simulink model "CompleteEngineModel_turbo"  (R2020a)
settings: Solver=ode23tb  StartTime=0  StopTime=600  MaxStep=0.4  RelTol=1e-6  AbsTol=1e-6  EnableMultiTasking=on
values from neighbouring files (symbols this model uses):
  A_eff_const = inv(A'*A)*A'*B    [Init_Project1.m]
  A_max_wg = 0.035^2/4*pi    (= 0.000962112750162)    [Init_Project1.m]    (also in Project2B.m = 0.000314159265359)
  AFs = EngineMap.airfuel.AFs    [Init_Project1.m]    (also in Project1b.m = 14)
  alpha_REF_manual = 0    [Init_Project1.m]    (also in Project2B.m)
  alphaEND = alphaINI    (= 0)    [Init_Project1.m]
  alphaINI = 0.0    (= 0)    [Init_Project1.m]
  alphaST = 30    [Init_Project1.m]
  Boost_control = 0    [Init_Project1.m]    (also in Project2B.m = 1)
  BSR_max = k(2)    [Project2A.m]
  C_d = x(3)    [Init_Project1.m]
  C_P0 = k(1)    [Project2A.m]
  C_P1 = k(2)    [Project2A.m]
  c_r1 = x(1)    [Init_Project1.m]
  c_r2 = x(2)    [Init_Project1.m]
  c_tc_fric = 1e-6    (= 1e-06)    [Init_Project1.m]    (also in Project2B.m)
  Cd_wg = 0.8    [Init_Project1.m]    (also in Project2B.m = 0.9)
  cp_air = gamma_air*cv_air    [Init_Project1.m]    (also in Project2A.m = 980)
  cp_exh = gamma_exh*cv_exh    [Init_Project1.m]    (also in Project2A.m = 1213.3)
  dP_thrREF = 10e3    (= 10000)    [Project2B.m]
  eta_c_max = k(1)    [Project2A.m]
  eta_t_max = k(1)    [Project2A.m]
  eta_vol_model = Intake_mainfold_const(1) + Intake_mainfold_const(2).*sqrt(p_im) + Intake_mainfold_const(3).*sqrt(N)    [Init_Project1.m]
  etaCmin = min(etaC/2)    [Project2A.m]
  etaTmin = min(turb.etaT)/2    [Project2A.m]
  Exhaust_flow_const = inv(A'*A)*A'*B    [Init_Project1.m]
  FMEP_const = inv(A'*A)*A'*B    [Init_Project1.m]
  Fuel_injection_const = inv(A'*A)*A'*B    [Init_Project1.m]
  gamma_air = EngineMap.airfuel.gamma_air    [Init_Project1.m]    (also in Project2A.m = 1.4)
  gamma_exh = EngineMap.airfuel.gamma_exh    [Init_Project1.m]    (also in Project2A.m = 1.3)
  Intake_mainfold_const = inv(A'*A)*A'*B    [Init_Project1.m]
  J_tc = 2.55e-5    (= 2.55e-05)    [Init_Project1.m]    (also in Project2B.m = 1e-05)
  k_0 = k(1)    [Project2A.m]
  k_1 = k(2)    [Project2A.m]
  KiDriver = 0.02    [Init_Project1.m]    (also in Project2B.m = 0.05)
  KpDriver = 0.04    [Init_Project1.m]    (also in Project2B.m = 0.8)
  KpThr = 1e-6    (= 1e-06)    [Init_Project1.m]    (also in Project2B.m)
  KpWg = 1e-6    (= 1e-06)    [Init_Project1.m]    (also in Project2B.m = 5e-06)
  m_dot_c_Corr_at = k(2)    [Project2A.m]
  m_dot_cCorr_max = k(2)    [Project2A.m]
  n_cyl = EngineMap.engine.n_cyl    [Init_Project1.m]    (also in Project2A.m)
  N_e_manual = 0    [Init_Project1.m]    (also in Project2B.m = 1)
  N_e_step = 1    [Init_Project1.m]    (also in Project2B.m)
  n_r = EngineMap.engine.n_r    [Init_Project1.m]    (also in Project2A.m; Project2B.m = 2)
  NEND = NINI    (= 2000)    [Init_Project1.m]    (also in Project2B.m = 2500)
  NeRampInit = 800    [Init_Project1.m]    (also in Project2B.m)
  NeSlope = 1    [Init_Project1.m]    (also in Project2B.m)
  NeST = 30    [Init_Project1.m]
  NINI = 2000    [Init_Project1.m]    (also in Project2B.m = 2500)
  p01 = comp.p01    [Project2A.m]
  p_amb = max(EngineMap.p_af)    [Init_Project1.m]
  pCref = comp.pCref    [Project2A.m]
  pedEND = 1.0    (= 1)    [Init_Project1.m]    (also in Project2B.m)
  pedINI = 0.2    [Init_Project1.m]    (also in Project2B.m = 0)
  pedPos_manual = 0    [Init_Project1.m]    (also in Project2B.m = 1)
  pedST = 30    [Init_Project1.m]    (also in Project2B.m)
  PiC_at = k(3)    [Project2A.m]
  Psi_max = k(1)    [Project2A.m]
  Q11 = k(4)    [Project2A.m]
  Q12 = k(5)    [Project2A.m]
  Q22 = k(6)    [Project2A.m]
  q_LHV = EngineMap.airfuel.q_LHV    [Init_Project1.m]
  R_air = EngineMap.airfuel.R_air    [Init_Project1.m]
  r_c = EngineMap.engine.r_c    [Init_Project1.m]    (also in Project1b.m = pCylHigh.r_c)
  R_exh = EngineMap.airfuel.R_exh    [Init_Project1.m]
  rComp = dComp/2    (= 0.028)    [Project2A.m]
  rho_air = p_amb/(R_air*T_amb)    [Init_Project1.m]
  rTurb = dTurb/2    (= 0.0261)    [Project2A.m]
  T01 = comp.T01    [Project2A.m]
  T_amb = mean(EngineMap.T_af)    [Init_Project1.m]
  T_bef_thr = EngineMap.T_bef_thr    [Init_Project1.m]
  T_es = EngineMap.T_es    [Init_Project1.m]
  T_ic = mean(T_bef_thr)    [Init_Project1.m]    (also in Project2B.m = T_im)
  T_im = EngineMap.T_im    [Init_Project1.m]    (also in Project1b.m = pCylHigh.T_im)
  tau_d = 0.069    [Init_Project1.m]
  tau_mix = 0.085    [Init_Project1.m]
  tau_th = 0.04    [Init_Project1.m]
  tau_wg = 0.1    [Init_Project1.m]    (also in Project2B.m)
  TCref = comp.TCref    [Project2A.m]
  Temp_const = inv(A'*A)*A'*B    [Init_Project1.m]
  TiThr = 0.1    [Init_Project1.m]    (also in Project2B.m = 0.4)
  TiWg = 4    [Init_Project1.m]    (also in Project2B.m = 7)
  V_D = EngineMap.engine.V_D    [Init_Project1.m]    (also in Project2B.m = n_cyl*V_d)
  V_d = 2*a*pi*B^2/4    [Init_Project1.m]    (also in Project2A.m; Project2B.m = B^2/4*pi*s)
  V_em = EngineMap.engine.V_em    [Init_Project1.m]
  V_es = EngineMap.engine.V_es    [Init_Project1.m]
  V_ic = 10e-3    (= 0.01)    [Init_Project1.m]    (also in Project2B.m)
  V_im = EngineMap.engine.V_im    [Init_Project1.m]
  VehicleArea = 2.0    (= 2)    [Init_Project1.m]
  VehicleMass = 1520    [Init_Project1.m]
  wg_REF_manual = 0    [Init_Project1.m]    (also in Project2B.m)
  wgEND = wgINI    (= 100)    [Init_Project1.m]
  wgINI = 100    [Init_Project1.m]
  wgST = 30    [Init_Project1.m]
  WheelRadius = 0.3    [Init_Project1.m]
undefined symbols (not defined in the file or in its folder): Newton, Raphson, TqEvsNe
libraries: simulink x2
(part 2 of 2)

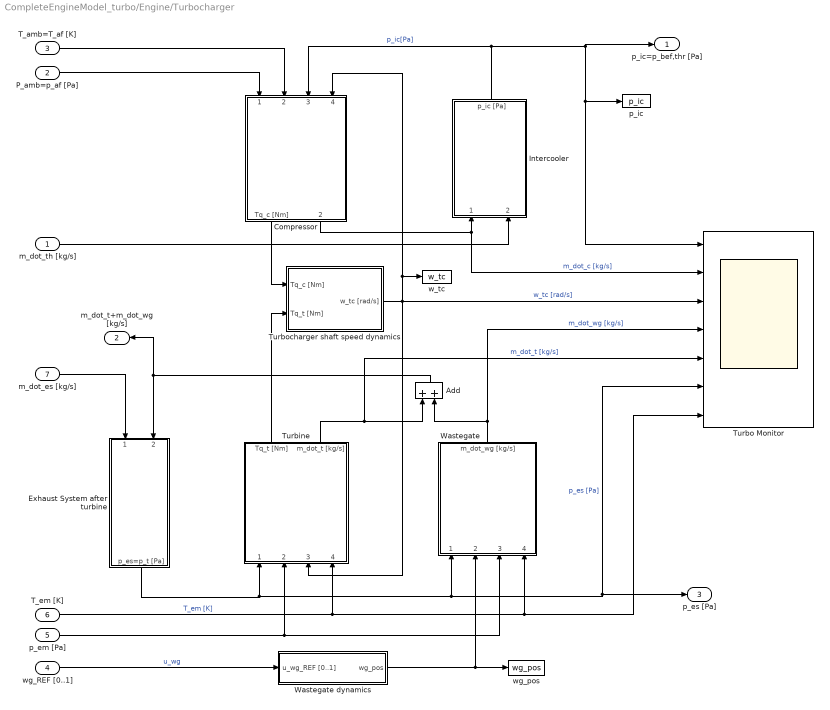
== system CompleteEngineModel_turbo/Engine/Turbocharger ==
  m_dot_th [kg/s] : Inport
  "P_amb=p_af [Pa] " : Inport  Port=2
  T_amb=T_af [K] : Inport  Port=3
  wg_REF [0..1] : Inport  Port=4
  p_em [Pa] : Inport  Port=5
  T_em [K] : Inport  Port=6
  m_dot_es [kg/s] : Inport  Port=7
  Add : Sum
  Compressor : Subsystem
  Exhaust System after turbine : Subsystem
  Intercooler : Subsystem
  Turbine : Subsystem
  Turbo Monitor : Scope  NumInputPorts=7
  Turbocharger shaft speed dynamics : Subsystem
  Wastegate : Subsystem
  Wastegate dynamics : Subsystem
  p_ic : ToWorkspace  VariableName=p_ic  SampleTime=-1
  w_tc : ToWorkspace  VariableName=w_tc  SampleTime=-1
  wg_pos : ToWorkspace  VariableName=wg_pos  SampleTime=-1
  p_ic=p_bef,thr [Pa] : Outport
  m_dot_t+m_dot_wg [kg/s] : Outport  Port=2
  p_es [Pa] : Outport  Port=3
  wires:
  Turbocharger shaft speed dynamics/1(w_tc [rad/s]) -> w_tc/1, Compressor/4(w_tc [rad/s]), Turbine/3(w_tc [rad/s]), Turbo Monitor/3  "w_tc [rad/s]"
  Wastegate dynamics/1(wg_pos) -> Wastegate/2(wg_pos [0..1]), wg_pos/1
  wg_REF [0..1]/1 -> Wastegate dynamics/1(u_wg_REF [0..1])  "u_wg"
  Compressor/2(m_dot_c [kg/s]) -> Turbo Monitor/2, Intercooler/1(Flow in [kg/s])  "m_dot_c [kg/s]"
  Intercooler/1(p_ic [Pa]) -> Compressor/3(p_ic [Pa]), p_ic/1, Turbo Monitor/1, p_ic=p_bef,thr [Pa]/1  "p_ic[Pa]"
  Compressor/1(Tq_c [Nm]) -> Turbocharger shaft speed dynamics/1(Tq_c [Nm])
  Turbine/1(Tq_t [Nm]) -> Turbocharger shaft speed dynamics/2(Tq_t [Nm])
  T_amb=T_af [K]/1 -> Compressor/2(T_af [K])
  "P_amb=p_af [Pa] "/1 -> Compressor/1(p_amb [Pa])
  m_dot_th [kg/s]/1 -> Intercooler/2(Flow  out [kg/s])
  Exhaust System after turbine/1(p_es=p_t [Pa]) -> Turbine/1("p_es [Pa] "), Wastegate/1(p_es [Pa]), p_es [Pa]/1, Turbo Monitor/6  "p_es [Pa]"
  p_em [Pa]/1 -> Wastegate/3(p_em [Pa]), Turbine/2(p_em [Pa])
  Turbine/2(m_dot_t [kg/s]) -> Turbo Monitor/5, Add/1  "m_dot_t [kg/s]"
  Add/1 -> Exhaust System after turbine/2(Flow in [kg/s]), m_dot_t+m_dot_wg [kg/s]/1
  m_dot_es [kg/s]/1 -> Exhaust System after turbine/1(Flow out [kg/s])
  T_em [K]/1 -> Wastegate/4(T_em [K]), Turbo Monitor/7, Turbine/4(T_em [K])  "T_em [K]"
  Wastegate/1(m_dot_wg [kg/s]) -> Add/2, Turbo Monitor/4  "m_dot_wg [kg/s]"

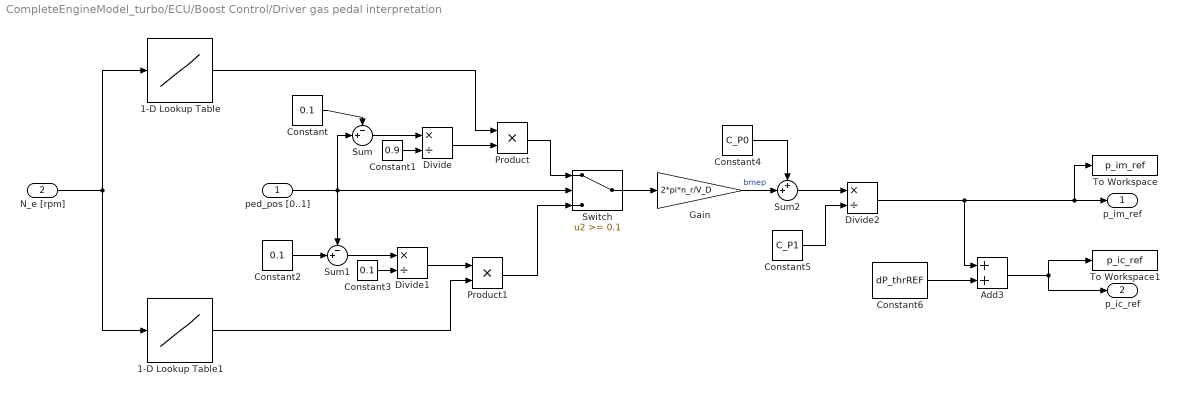
== system CompleteEngineModel_turbo/ECU/Boost Control/Driver gas pedal interpretation ==
  ped_pos [0..1] : Inport
  N_e [rpm] : Inport  Port=2
  1-D Lookup Table : Lookup_n-D  NumberOfTableDimensions=1  BreakpointsForDimension1=TqEvsNe.Ne  Table=TqEvsNe.TqMAX  InternalRulePriority=Speed  RndMeth=Simplest  InputSameDT=on
  1-D Lookup Table1 : Lookup_n-D  NumberOfTableDimensions=1  BreakpointsForDimension1=TqEvsNe.Ne  Table=TqEvsNe.TqMIN  InternalRulePriority=Speed  RndMeth=Simplest  InputSameDT=on
  Add3 : Sum
  Constant : Constant  Value=0.1
  Constant1 : Constant  Value=0.9
  Constant2 : Constant  Value=0.1
  Constant3 : Constant  Value=0.1
  Constant4 : Constant  Value=C_P0
  Constant5 : Constant  Value=C_P1
  Constant6 : Constant  Value=dP_thrREF
  Divide : Product  Inputs=*/
  Divide1 : Product  Inputs=*/
  Divide2 : Product  Inputs=*/
  Gain : Gain  Gain=2*pi*n_r/V_D
  Product : Product
  Product1 : Product
  Sum : Sum  Inputs=-+|
  Sum1 : Sum  Inputs=-+|
  Sum2 : Sum  Inputs=++|
  Switch : Switch  Threshold=0.1
  To Workspace : ToWorkspace  VariableName=p_im_ref  SaveFormat=Structure With Time  SampleTime=-1
  To Workspace1 : ToWorkspace  VariableName=p_ic_ref  SaveFormat=Structure With Time  SampleTime=-1
  p_im_ref : Outport
  p_ic_ref : Outport  Port=2
  wires:
  Add3/1 -> p_ic_ref/1, To Workspace1/1
  Constant6/1 -> Add3/2
  N_e [rpm]/1 -> 1-D Lookup Table1/1, 1-D Lookup Table/1
  ped_pos [0..1]/1 -> Switch/2, Sum1/1, Sum/2
  Constant/1 -> Sum/1
  Sum/1 -> Divide/1
  Constant1/1 -> Divide/2
  Divide/1 -> Product/2
  Product/1 -> Switch/1
  Constant2/1 -> Sum1/2
  Constant3/1 -> Divide1/2
  Sum1/1 -> Divide1/1
  Divide1/1 -> Product1/1
  Product1/1 -> Switch/3
  Switch/1 -> Gain/1
  Gain/1 -> Sum2/2  "bmep"
  Constant4/1 -> Sum2/1
  Sum2/1 -> Divide2/1
  Constant5/1 -> Divide2/2
  Divide2/1 -> Add3/1, To Workspace/1, p_im_ref/1
  1-D Lookup Table1/1 -> Product1/2
  1-D Lookup Table/1 -> Product/1

== system CompleteEngineModel_turbo/ECU/Boost Control/Throttle Feed Forward  ==
  p_imREF [Pa] : Inport
  N_e [rpm] : Inport  Port=2
  p_icACT [Pa] : Inport  Port=3
  Constant : Constant  Value=R_air*T01
  Cylinder air flow REF : Subsystem
  Divide : Product  Inputs=*/
  Divide1 : Product  Inputs=*/
  Gain : Gain  Gain=p01
  Max : MinMax  Function=max  Inputs=2
  Product : Product
  Psi(PI) : Subsystem
  Sqrt : Sqrt  SaturateOnIntegerOverflow=on
  Subsystem : Subsystem
  rpm2rps : Gain  Gain=1/60  SaturateOnIntegerOverflow=on  OutDataTypeStr=Inherit: Same as input  ParamDataTypeStr=Inherit: Same as input
  alpha_thrFF [0..1] : Outport
  wires:
  p_imREF [Pa]/1 -> Cylinder air flow REF/1(p_im_REF), Divide/1, Max/1
  N_e [rpm]/1 -> rpm2rps/1
  p_icACT [Pa]/1 -> Max/2
  Cylinder air flow REF/1(m_dot_ac_REF) -> Product/2
  Divide/1 -> Psi(PI)/1(PI)  "PI_REF"
  Max/1 -> Divide/2
  rpm2rps/1 -> Cylinder air flow REF/2(N [rps])
  Psi(PI)/1(Psi) -> Gain/1  "Psi_REF"
  Subsystem/1(alpha_thr_REF) -> alpha_thrFF [0..1]/1
  Constant/1 -> Sqrt/1
  Sqrt/1 -> Product/1
  Product/1 -> Divide1/1
  Divide1/1 -> Subsystem/1(A_thr_eff_REF)
  Gain/1 -> Divide1/2

== system CompleteEngineModel_turbo/ECU/Boost Control/Throttle Feedback including anti-windup ==
  p_imREF [Pa] : Inport
  p_imACT [Pa] : Inport  Port=2
  alpha_thrREFsat [0..1] : Inport  Port=3
  alpha_thrREF [0..1] : Inport  Port=4
  Integrator1 : Integrator  UpperSaturationLimit=5  LowerSaturationLimit=-5
  Subtract1 : Sum
  Subtract2 : Sum  Inputs=+-
  Subtract3 : Sum  Inputs=-+
  Subtract4 : Sum
  u_FB_wg_Kp : Gain  Gain=KpThr
  u_FB_wg_Kp1 : Gain  Gain=KpThr/TiThr
  u_FB_wg_Kp2 : Gain  Gain=1/TiThr
  alpha_thrFB [0..1] : Outport
  wires:
  p_imACT [Pa]/1 -> Subtract3/1
  p_imREF [Pa]/1 -> Subtract3/2
  Subtract3/1 -> u_FB_wg_Kp/1, u_FB_wg_Kp1/1  "controller error"
  u_FB_wg_Kp/1 -> Subtract4/1
  Subtract4/1 -> alpha_thrFB [0..1]/1
  u_FB_wg_Kp1/1 -> Subtract1/1
  alpha_thrREFsat [0..1]/1 -> Subtract2/1
  alpha_thrREF [0..1]/1 -> Subtract2/2
  Subtract2/1 -> u_FB_wg_Kp2/1
  u_FB_wg_Kp2/1 -> Subtract1/2
  Subtract1/1 -> Integrator1/1
  Integrator1/1 -> Subtract4/2

== system CompleteEngineModel_turbo/ECU/Boost Control/Waste-gate Feedback including anti-windup1 ==
  p_icREF [Pa] : Inport
  p_icACT [Pa] : Inport  Port=2
  wgREFsat [0..1] : Inport  Port=3
  wgREF [0..1] : Inport  Port=4
  Integrator1 : Integrator  InitialCondition=0.3
  Subtract1 : Sum
  Subtract2 : Sum  Inputs=+-
  Subtract3 : Sum  Inputs=+-
  Subtract4 : Sum
  Tracking : Gain  Gain=1/TiWg
  u_FB_wg_Integral : Gain  Gain=KpWg/TiWg
  u_FB_wg_Proportional : Gain  Gain=KpWg
  wgFB [0..1] : Outport
  wires:
  Integrator1/1 -> Subtract4/2
  Subtract1/1 -> Integrator1/1
  Tracking/1 -> Subtract1/2
  Subtract2/1 -> Tracking/1
  wgREF [0..1]/1 -> Subtract2/2
  wgREFsat [0..1]/1 -> Subtract2/1
  u_FB_wg_Integral/1 -> Subtract1/1
  Subtract4/1 -> wgFB [0..1]/1
  u_FB_wg_Proportional/1 -> Subtract4/1
  Subtract3/1 -> u_FB_wg_Proportional/1, u_FB_wg_Integral/1  "controller error"
  p_icACT [Pa]/1 -> Subtract3/1
  p_icREF [Pa]/1 -> Subtract3/2

== system CompleteEngineModel_turbo/ECU/Fuel Cont/m_dot_ac_system ==
  p_im : Inport
  N : Inport  Port=2
  Abs : Abs
  Abs1 : Abs
  Constant : Constant  Value=mean(eta_vol_model)
  Divide : Product  Inputs=*/
  Product : Product  Inputs=5
  Product1 : Product  Inputs=3
  R : Constant  Value=R_air
  T_im : Constant  Value=mean(T_im)
  V_d : Constant  Value=V_d
  n_cyl : Constant  Value=n_cyl
  n_r : Constant  Value=n_r
  m_dot_ac : Outport
  wires:
  V_d/1 -> Product/3
  n_cyl/1 -> Product/4
  Product/1 -> Divide/1
  n_r/1 -> Product1/1
  T_im/1 -> Product1/2
  R/1 -> Product1/3
  Product1/1 -> Divide/2
  Divide/1 -> m_dot_ac/1
  N/1 -> Abs1/1
  Abs1/1 -> Product/2
  p_im/1 -> Abs/1
  Abs/1 -> Product/5
  Constant/1 -> Product/1

== system CompleteEngineModel_turbo/Engine/Cylinder/m_dot_ac_system ==
  p_im : Inport
  N : Inport  Port=2
  Abs : Abs
  Abs1 : Abs
  Divide : Product  Inputs=*/
  Product : Product  Inputs=5
  Product1 : Product  Inputs=3
  R : Constant  Value=R_air
  Sqrt : Sqrt  SaturateOnIntegerOverflow=on
  Sqrt1 : Sqrt  SaturateOnIntegerOverflow=on
  Sum : Sum  Inputs=|++
  Sum1 : Sum  Inputs=|++
  T_im : Constant  Value=mean(T_im)
  V_d : Constant  Value=V_d
  c0 : Constant  Value=Intake_mainfold_const(1)
  c1 : Gain  Gain=Intake_mainfold_const(2)
  c2 : Gain  Gain=Intake_mainfold_const(3)
  n_cyl : Constant  Value=n_cyl
  n_r : Constant  Value=n_r
  m_dot_ac : Outport
  wires:
  Sum1/1 -> Product/1  "eta_vol"
  c2/1 -> Sum/2
  Sum/1 -> Sum1/1
  c1/1 -> Sum/1
  c0/1 -> Sum1/2
  Sqrt/1 -> c1/1
  Sqrt1/1 -> c2/1
  V_d/1 -> Product/3
  n_cyl/1 -> Product/4
  Product/1 -> Divide/1
  n_r/1 -> Product1/1
  T_im/1 -> Product1/2
  R/1 -> Product1/3
  Product1/1 -> Divide/2
  Divide/1 -> m_dot_ac/1
  N/1 -> Abs1/1
  Abs1/1 -> Product/2, Sqrt1/1
  p_im/1 -> Abs/1
  Abs/1 -> Sqrt/1, Product/5

== system CompleteEngineModel_turbo/Engine/Lambda sensor/If Action Subsystem ==
  In1 : Inport
  Action Port : ActionPort  ActionPortLabel=if(u1 > 1)
  Out1 : Outport
  wires:
  In1/1 -> Out1/1

== system CompleteEngineModel_turbo/Engine/Lambda sensor/If Action Subsystem1 ==
  In1 : Inport
  Action Port : ActionPort  ActionPortLabel=elseif(u1 == 1)
  Out1 : Outport
  wires:
  In1/1 -> Out1/1

== system CompleteEngineModel_turbo/Engine/Lambda sensor/If Action Subsystem2 ==
  In1 : Inport
  Action Port : ActionPort  ActionPortLabel=elseif( u1 < 1)
  Out1 : Outport
  wires:
  In1/1 -> Out1/1

== system CompleteEngineModel_turbo/Engine/Throttle /A_eff ==
  alpha : Inport
  Product : Product
  Sum : Sum  Inputs=|++
  Sum1 : Sum  Inputs=|++
  a0 : Constant  Value=A_eff_const(1)
  a1 : Gain  Gain=A_eff_const(2)
  a2 : Gain  Gain=A_eff_const(3)
  A_eff : Outport
  wires:
  alpha/1 -> Product/2, Product/1, a1/1
  a1/1 -> Sum/1  "a_1*alpha"
  a2/1 -> Sum/2  "a_2*alpha^2"
  a0/1 -> Sum1/2
  Product/1 -> a2/1  "alpha^2"
  Sum/1 -> Sum1/1  "a1*alpha + a2*alpha^2"
  Sum1/1 -> A_eff/1  "A_eff"

== system CompleteEngineModel_turbo/Engine/Throttle /Psi(PI) ==
  PI : Inport
  (g+1)/g : Constant  Value=(gamma_air+1)/gamma_air
  2/g : Constant  Value=2/gamma_air
  2g/(g-1) : Constant  Value=(2*gamma_air)/(gamma_air-1)
  Math Function : Math  Operator=pow  SignedPower=on  SaturateOnIntegerOverflow=on
  Math Function1 : Math  Operator=pow  SignedPower=on  SaturateOnIntegerOverflow=on
  MinMax : MinMax  Function=max  Inputs=2
  PI critical (2/(g+1))^(g/(g-1)) : Constant  Value=(2/(gamma_air+1))^(gamma_air/(gamma_air-1))
  Product : Product  RndMeth=Zero
  Sqrt : Sqrt  AlgorithmType=Newton-Raphson  SaturateOnIntegerOverflow=on
  Subtract : Sum  Inputs=+-
  "[0,1]" : Saturate  UpperLimit=1  LowerLimit=0
  Psi : Outport
  wires:
  PI/1 -> "[0,1]"/1  "PI"
  PI critical (2/(g+1))^(g/(g-1))/1 -> MinMax/2
  MinMax/1 -> Math Function/1, Math Function1/1  "PIlim"
  2/g/1 -> Math Function/2
  (g+1)/g/1 -> Math Function1/2
  "[0,1]"/1 -> MinMax/1
  Math Function/1 -> Subtract/1
  Math Function1/1 -> Subtract/2
  Subtract/1 -> Product/1
  2g/(g-1)/1 -> Product/2
  Product/1 -> Sqrt/1
  Sqrt/1 -> Psi/1  "Psi"

== system CompleteEngineModel_turbo/Engine/Turbocharger/Compressor ==
  note: You are expected to implement your model here, only for Project 2!
  p_amb [Pa] : Inport
  T_af [K] : Inport  Port=2
  p_ic [Pa] : Inport  Port=3
  w_tc [rad/s] : Inport  Port=4
  PiCmax : Subsystem
  Product4 : Product  Inputs=*/  RndMeth=Zero
  Tc : Subsystem
  Tq_c : Subsystem
  WcCorr2Wc : Subsystem
  etaC : Subsystem
  m_dot_cCorr : Subsystem
  Tq_c [Nm] : Outport
  m_dot_c [kg/s] : Outport  Port=2
  wires:
  w_tc [rad/s]/1 -> PiCmax/2(w_tc), Tq_c/4(w_tc)
  p_ic [Pa]/1 -> Product4/1
  p_amb [Pa]/1 -> WcCorr2Wc/1(p_amb), Product4/2
  T_af [K]/1 -> PiCmax/1(Tamb), WcCorr2Wc/2(T_amb), Tc/3(Tamb), Tq_c/3(Tamb)
  WcCorr2Wc/1(m_dot_c) -> m_dot_c [kg/s]/1, Tq_c/1(m_dot_c)
  Product4/1 -> etaC/2(PiC), Tc/2(PiC), m_dot_cCorr/2(PiC)  "PiC"
  m_dot_cCorr/1(m_dot_cCorr) -> WcCorr2Wc/3(m_dot_cCorr), etaC/1(m_dot_cCorr)
  Tc/1(T02) -> Tq_c/2(T02)
  Tq_c/1(Tq_c) -> Tq_c [Nm]/1
  PiCmax/1(PiCmax) -> m_dot_cCorr/1(PiCmax)
  etaC/1(etaC) -> Tc/1(etaC)

== system CompleteEngineModel_turbo/Engine/Turbocharger/Exhaust System after turbine ==
  Flow out [kg/s] : Inport
  Flow in [kg/s] : Inport  Port=2
  Integrator : Integrator  InitialCondition=103e3
  Product : Product  Inputs=***/  SaturateOnIntegerOverflow=on  OutDataTypeStr=Inherit: Same as first input
  R : Constant  Value=R_exh
  Sum : Sum  Inputs=|+-  SaturateOnIntegerOverflow=on
  T_t : Constant  Value=mean(T_es)
  V_es : Constant  Value=V_es
  p_es=p_t [Pa] : Outport
  wires:
  V_es/1 -> Product/4
  Sum/1 -> Product/1
  T_t/1 -> Product/3
  R/1 -> Product/2
  Flow out [kg/s]/1 -> Sum/2
  Flow in [kg/s]/1 -> Sum/1
  Product/1 -> Integrator/1
  Integrator/1 -> p_es=p_t [Pa]/1

== system CompleteEngineModel_turbo/Engine/Turbocharger/Intercooler ==
  Flow in [kg/s] : Inport
  Flow  out [kg/s] : Inport  Port=2
  Integrator : Integrator  InitialCondition=p_amb  LowerSaturationLimit=0
  Product : Product  Inputs=***/  SaturateOnIntegerOverflow=on  OutDataTypeStr=Inherit: Same as first input
  R : Constant  Value=R_air
  Sum : Sum  Inputs=|+-  SaturateOnIntegerOverflow=on
  T_ic : Constant  Value=mean(T_ic)
  V_ic : Constant  Value=V_ic
  p_ic [Pa] : Outport
  wires:
  Integrator/1 -> p_ic [Pa]/1
  Flow in [kg/s]/1 -> Sum/1
  Flow  out [kg/s]/1 -> Sum/2
  R/1 -> Product/2
  T_ic/1 -> Product/3
  Sum/1 -> Product/1
  V_ic/1 -> Product/4
  Product/1 -> Integrator/1

== system CompleteEngineModel_turbo/Engine/Turbocharger/Turbine ==
  note: You are expected to implement your model here, only for Project 2!
  "p_es [Pa] " : Inport
  p_em [Pa] : Inport  Port=2
  w_tc [rad/s] : Inport  Port=3
  T_em [K] : Inport  Port=4
  BSR : Subsystem
  PiT : Subsystem
  TFP2Wt : Subsystem
  TFPmod : Subsystem
  Tq_t : Subsystem
  Tt : Subsystem
  etaT : Subsystem
  Tq_t [Nm] : Outport
  m_dot_t [kg/s] : Outport  Port=2
  wires:
  w_tc [rad/s]/1 -> BSR/3(w_tc [rad/s]), Tq_t/4(w_tc)
  "p_es [Pa] "/1 -> PiT/2(p_es)  "p_t [Pa]"
  p_em [Pa]/1 -> PiT/1(p_em), TFP2Wt/1(p_em [Pa])
  PiT/1(PiT) -> TFPmod/1(PiT), BSR/2(PiT), Tt/3(PiT)
  TFPmod/1(TFPmod) -> TFP2Wt/2(TFP)
  TFP2Wt/1(m_dot_t) -> m_dot_t [kg/s]/1, Tq_t/1(m_dot_t)
  BSR/1(BSR) -> etaT/1(BSR)
  T_em [K]/1 -> TFP2Wt/3(T_em), BSR/1(T_em), Tq_t/2(T_em), Tt/1(T_em)
  etaT/1(etaT) -> Tt/2(etaT)
  Tt/1(T04) -> Tq_t/3(T04)
  Tq_t/1(Tq_t) -> Tq_t [Nm]/1

== system CompleteEngineModel_turbo/Engine/Turbocharger/Turbocharger shaft speed dynamics ==
  Tq_c [Nm] : Inport
  Tq_t [Nm] : Inport  Port=2
  Gain : Gain  Gain=1 / J_tc
  Gain1 : Gain  Gain=c_tc_fric
  Gain2 : Gain  Gain=60/(2*pi)
  Integrator with lower saturation : Integrator  InitialCondition=25e3/30*pi  LimitOutput=on  LowerSaturationLimit="5e3 /  30 * pi"
  Sum : Sum  Inputs=+--
  To Workspace : ToWorkspace  VariableName=turbo_speed  SampleTime=-1
  w_tc [rad/s] : Outport
  wires:
  Integrator with lower saturation/1 -> Gain1/1, Gain2/1, w_tc [rad/s]/1
  Gain/1 -> Integrator with lower saturation/1
  Tq_t [Nm]/1 -> Sum/1
  Tq_c [Nm]/1 -> Sum/2
  Gain1/1 -> Sum/3
  Sum/1 -> Gain/1
  Gain2/1 -> To Workspace/1

== system CompleteEngineModel_turbo/Engine/Turbocharger/Wastegate ==
  note: You are expected to implement your model here, only for Project 2!
  p_es [Pa] : Inport
  wg_pos [0..1] : Inport  Port=2
  p_em [Pa] : Inport  Port=3
  T_em [K] : Inport  Port=4
  A_max_wg : Constant  Value=A_max_wg
  Cd_wg : Constant  Value=Cd_wg
  Divide : Product  Inputs=*/
  Divide1 : Product  Inputs=***/
  Product1 : Product  Inputs=3  RndMeth=Zero
  Product2 : Product  RndMeth=Zero
  Psi(PI) : Subsystem
  R : Constant  Value=R_exh
  Saturation : Saturate  UpperLimit=1  LowerLimit=0
  Scope1 : Scope  NumInputPorts=2
  Scope2 : Scope
  Scope3 : Scope
  Sqrt : Sqrt  AlgorithmType=Newton-Raphson  SaturateOnIntegerOverflow=on
  m_dot_wg [kg/s] : Outport
  wires:
  Divide1/1 -> Scope2/1, m_dot_wg [kg/s]/1
  p_em [Pa]/1 -> Divide/2, Divide1/2
  Divide/1 -> Psi(PI)/1(PI)  "PI"
  Product1/1 -> Divide1/3  "Aeff"
  Product2/1 -> Scope3/1, Sqrt/1  "RT"
  Sqrt/1 -> Divide1/4  "sqrt(RT)"
  Psi(PI)/1(Psi) -> Divide1/1  "Psi"
  R/1 -> Product2/1  "R"
  T_em [K]/1 -> Product2/2  "T"
  wg_pos [0..1]/1 -> Scope1/1, Saturation/1
  A_max_wg/1 -> Product1/2
  Cd_wg/1 -> Product1/3
  Saturation/1 -> Scope1/2, Product1/1
  p_es [Pa]/1 -> Divide/1

== system CompleteEngineModel_turbo/Engine/Turbocharger/Wastegate dynamics ==
  note: You are expected to implement your model here, only for Project 2!
  u_wg_REF [0..1] : Inport
  Gain : Gain  Gain=1 / tau_wg
  Integrator : Integrator
  Saturation : Saturate  UpperLimit=1  LowerLimit=0
  Sum : Sum  Inputs=|+-
  wg_pos : Outport
  wires:
  u_wg_REF [0..1]/1 -> Saturation/1
  Gain/1 -> Integrator/1
  Sum/1 -> Gain/1
  Saturation/1 -> Sum/1
  Integrator/1 -> wg_pos/1, Sum/2

== system CompleteEngineModel_turbo/ECU/Boost Control/Throttle Feed Forward /Cylinder air flow REF ==
  p_im_REF : Inport
  N [rps] : Inport  Port=2
  Volymetrisk effektivitet : Subsystem
  m_dot_ac_system : Subsystem
  m_dot_ac_REF : Outport
  wires:
  p_im_REF/1 -> Volymetrisk effektivitet/1(" p_im"), m_dot_ac_system/1(p_im_REF)
  N [rps]/1 -> m_dot_ac_system/3(N), Volymetrisk effektivitet/2(N)
  Volymetrisk effektivitet/1(eta_vol) -> m_dot_ac_system/2(Eta_vol_REF)
  m_dot_ac_system/1(m_dot_ac) -> m_dot_ac_REF/1

== system CompleteEngineModel_turbo/ECU/Boost Control/Throttle Feed Forward /Psi(PI) ==
  PI : Inport
  (g+1)/g : Constant  Value=(gamma_air+1)/gamma_air
  2/g : Constant  Value=2/gamma_air
  2g/(g-1) : Constant  Value=(2*gamma_air)/(gamma_air-1)
  Display3 : Display
  Display4 : Display
  DivZeroProtect : MinMax  Function=max  Inputs=2
  Math Function : Math  Operator=pow  SignedPower=on  SaturateOnIntegerOverflow=on
  Math Function1 : Math  Operator=pow  SignedPower=on  SaturateOnIntegerOverflow=on
  MinMax : MinMax  Function=max  Inputs=2
  PI critical (2/(g+1))^(g/(g-1)) : Constant  Value=(2/(gamma_air+1))^(gamma_air/(gamma_air-1))
  Product : Product  RndMeth=Zero
  Sqrt : Sqrt  AlgorithmType=Newton-Raphson  SaturateOnIntegerOverflow=on
  Subtract : Sum  Inputs=+-
  "[0,1]" : Saturate  UpperLimit=1  LowerLimit=0
  eps : Constant  Value=eps
  Psi : Outport
  wires:
  PI/1 -> "[0,1]"/1  "PI"
  PI critical (2/(g+1))^(g/(g-1))/1 -> MinMax/2
  MinMax/1 -> Math Function/1, Math Function1/1  "PIlim"
  2/g/1 -> Math Function/2
  (g+1)/g/1 -> Math Function1/2
  "[0,1]"/1 -> MinMax/1
  Math Function/1 -> Subtract/1
  Math Function1/1 -> Subtract/2
  Subtract/1 -> Product/1
  2g/(g-1)/1 -> Product/2
  Product/1 -> Sqrt/1
  Sqrt/1 -> Display3/1, DivZeroProtect/1  "Psi"
  eps/1 -> DivZeroProtect/2
  DivZeroProtect/1 -> Display4/1, Psi/1

== system CompleteEngineModel_turbo/ECU/Boost Control/Throttle Feed Forward /Subsystem ==
  A_thr_eff_REF : Inport
  Constant : Constant  Value=0
  Constant2 : Constant  Value=2*A_eff_const(3)
  Divide : Product  Inputs=*/
  Divide1 : Product  Inputs=*/
  Ev byt tecken : Gain
  Max : MinMax  Function=max  Inputs=2
  Saturation : Saturate  UpperLimit=A_max_wg  LowerLimit=0
  Sqrt : Sqrt  SaturateOnIntegerOverflow=on
  Square : Math  Operator=square  SaturateOnIntegerOverflow=on
  Sum : Sum  Inputs=|+-
  Sum2 : Sum  Inputs=|+-
  Sum3 : Sum  Inputs=|++
  a0 : Constant  Value=A_eff_const(1)
  a1 : Constant  Value=A_eff_const(2)
  a2 : Constant  Value=A_eff_const(3)
  alpha_thr_REF : Outport
  wires:
  a0/1 -> Sum2/2
  Sum2/1 -> Divide/1
  a2/1 -> Divide/2
  Divide/1 -> Sum3/1
  a1/1 -> Divide1/1
  Constant2/1 -> Divide1/2
  Divide1/1 -> Sum/2, Square/1
  Square/1 -> Sum3/2
  Sqrt/1 -> Ev byt tecken/1
  Sum/1 -> alpha_thr_REF/1
  Ev byt tecken/1 -> Sum/1
  Saturation/1 -> Sum2/1
  A_thr_eff_REF/1 -> Saturation/1
  Constant/1 -> Max/2
  Max/1 -> Sqrt/1
  Sum3/1 -> Max/1

== system CompleteEngineModel_turbo/Engine/Turbocharger/Compressor/PiCmax ==
  Tamb : Inport
  w_tc : Inport  Port=2
  Constant : Constant
  Constant1 : Constant  Value=(gamma_air) / (gamma_air - 1)
  Divide : Product  Inputs=*/
  Gain : Gain  Gain=rComp
  Gain1 : Gain  Gain=Psi_max
  Gain2 : Gain  Gain=2*cp_air
  Power : Math  Operator=pow  SaturateOnIntegerOverflow=on
  Square : Math  Operator=square  SaturateOnIntegerOverflow=on
  Sum : Sum  Inputs=++|
  PiCmax : Outport
  wires:
  w_tc/1 -> Gain/1
  Gain/1 -> Square/1  "u2"
  Square/1 -> Gain1/1
  Tamb/1 -> Gain2/1
  Constant/1 -> Sum/1
  Gain1/1 -> Divide/1
  Gain2/1 -> Divide/2
  Constant1/1 -> Power/2
  Power/1 -> PiCmax/1
  Divide/1 -> Sum/2
  Sum/1 -> Power/1

== system CompleteEngineModel_turbo/Engine/Turbocharger/Compressor/Tc ==
  etaC : Inport
  PiC : Inport  Port=2
  Tamb : Inport  Port=3
  Constant : Constant  Value=(gamma_air - 1) / gamma_air
  Constant1 : Constant
  Constant2 : Constant
  Divide : Product  Inputs=*/
  Power : Math  Operator=pow  SaturateOnIntegerOverflow=on
  Product : Product
  Sum : Sum  Inputs=|+-
  Sum1 : Sum  Inputs=|++
  T02 : Outport
  wires:
  Tamb/1 -> Product/2
  etaC/1 -> Divide/2
  PiC/1 -> Power/1
  Product/1 -> T02/1
  Constant/1 -> Power/2
  Power/1 -> Sum/1
  Constant1/1 -> Sum/2
  Sum/1 -> Divide/1
  Divide/1 -> Sum1/1
  Constant2/1 -> Sum1/2
  Sum1/1 -> Product/1

== system CompleteEngineModel_turbo/Engine/Turbocharger/Compressor/Tq_c ==
  m_dot_c : Inport
  T02 : Inport  Port=2
  Tamb : Inport  Port=3
  w_tc : Inport  Port=4
  Constant : Constant  Value=cp_air
  Divide : Product  Inputs=*/
  Product : Product  Inputs=3
  Sum : Sum  Inputs=|+-
  Tq_c : Outport
  wires:
  Tamb/1 -> Sum/2
  T02/1 -> Sum/1
  m_dot_c/1 -> Product/1
  w_tc/1 -> Divide/2
  Constant/1 -> Product/2
  Sum/1 -> Product/3
  Product/1 -> Divide/1
  Divide/1 -> Tq_c/1

== system CompleteEngineModel_turbo/Engine/Turbocharger/Compressor/WcCorr2Wc ==
  p_amb : Inport
  T_amb : Inport  Port=2
  m_dot_cCorr : Inport  Port=3
  Divide : Product  Inputs=*/
  Gain : Gain  Gain=1 / pCref
  Gain1 : Gain  Gain=1 / TCref
  Product : Product
  Sqrt : Sqrt  SaturateOnIntegerOverflow=on
  m_dot_c : Outport
  wires:
  Divide/1 -> m_dot_c/1
  T_amb/1 -> Gain1/1
  p_amb/1 -> Gain/1
  m_dot_cCorr/1 -> Product/1
  Gain1/1 -> Sqrt/1
  Gain/1 -> Product/2
  Product/1 -> Divide/1
  Sqrt/1 -> Divide/2

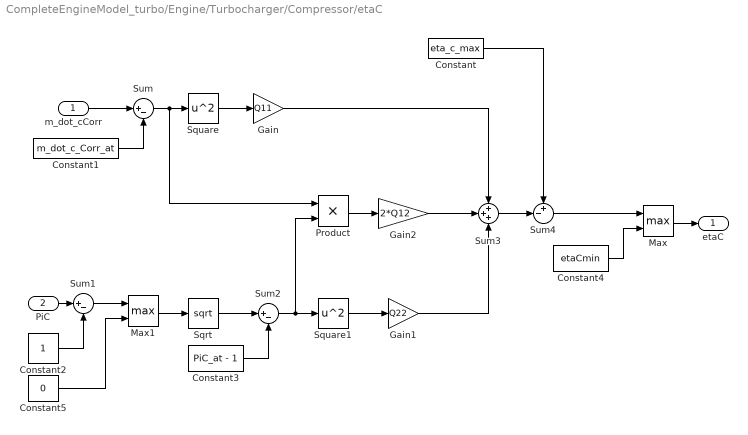
== system CompleteEngineModel_turbo/Engine/Turbocharger/Compressor/etaC ==
  m_dot_cCorr : Inport
  PiC : Inport  Port=2
  Constant : Constant  Value=eta_c_max
  Constant1 : Constant  Value=m_dot_c_Corr_at
  Constant2 : Constant
  Constant3 : Constant  Value=PiC_at - 1
  Constant4 : Constant  Value=etaCmin
  Constant5 : Constant  Value=0
  Gain : Gain  Gain=Q11
  Gain1 : Gain  Gain=Q22
  Gain2 : Gain  Gain=2*Q12
  Max : MinMax  Function=max  Inputs=2
  Max1 : MinMax  Function=max  Inputs=2
  Product : Product
  Sqrt : Sqrt  SaturateOnIntegerOverflow=on
  Square : Math  Operator=square  SaturateOnIntegerOverflow=on
  Square1 : Math  Operator=square  SaturateOnIntegerOverflow=on
  Sum : Sum  Inputs=|+-
  Sum1 : Sum  Inputs=|+-
  Sum2 : Sum  Inputs=|+-
  Sum3 : Sum  Inputs=+++
  Sum4 : Sum  Inputs=+-|
  etaC : Outport
  wires:
  Sum4/1 -> Max/1
  Constant4/1 -> Max/2
  Max/1 -> etaC/1
  m_dot_cCorr/1 -> Sum/1
  PiC/1 -> Sum1/1
  Constant1/1 -> Sum/2
  Sum/1 -> Product/1, Square/1
  Square/1 -> Gain/1
  Constant2/1 -> Sum1/2
  Sqrt/1 -> Sum2/1
  Constant3/1 -> Sum2/2
  Sum2/1 -> Product/2, Square1/1
  Square1/1 -> Gain1/1
  Product/1 -> Gain2/1
  Gain2/1 -> Sum3/2
  Gain/1 -> Sum3/1
  Gain1/1 -> Sum3/3
  Sum3/1 -> Sum4/2
  Constant/1 -> Sum4/1
  Constant5/1 -> Max1/2
  Max1/1 -> Sqrt/1
  Sum1/1 -> Max1/1

== system CompleteEngineModel_turbo/Engine/Turbocharger/Compressor/m_dot_cCorr ==
  PiCmax : Inport
  PiC : Inport  Port=2
  Constant : Constant
  Divide : Product  Inputs=*/
  Gain : Gain  Gain=m_dot_cCorr_max
  Sqrt : Sqrt  SaturateOnIntegerOverflow=on
  Square : Math  Operator=square  SaturateOnIntegerOverflow=on
  Sum : Sum  Inputs=+-|
  To Workspace1 : ToWorkspace  VariableName=m_dot_cCorr  SampleTime=-1
  m_dot_cCorr : Outport
  wires:
  Gain/1 -> To Workspace1/1, m_dot_cCorr/1
  PiCmax/1 -> Divide/2
  PiC/1 -> Divide/1
  Divide/1 -> Square/1
  Square/1 -> Sum/2
  Constant/1 -> Sum/1
  Sum/1 -> Sqrt/1
  Sqrt/1 -> Gain/1

== system CompleteEngineModel_turbo/Engine/Turbocharger/Turbine/BSR ==
  T_em : Inport
  PiT : Inport  Port=2
  w_tc [rad/s] : Inport  Port=3
  Constant : Constant  Value=(gamma_exh - 1) / gamma_exh
  Constant1 : Constant
  Divide : Product  Inputs=*/
  Gain : Gain  Gain=rTurb
  Gain1 : Gain  Gain=2*cp_exh
  Power : Math  Operator=pow  SaturateOnIntegerOverflow=on
  Product : Product
  Saturation : Saturate  UpperLimit=1  LowerLimit=0.1
  Sqrt : Sqrt  SaturateOnIntegerOverflow=on
  Sum : Sum  Inputs=+-|
  BSR : Outport
  wires:
  w_tc [rad/s]/1 -> Gain/1
  PiT/1 -> Power/1
  T_em/1 -> Product/2
  Divide/1 -> Saturation/1
  Saturation/1 -> BSR/1
  Constant/1 -> Power/2
  Power/1 -> Sum/2
  Constant1/1 -> Sum/1
  Sum/1 -> Product/1
  Product/1 -> Gain1/1
  Gain1/1 -> Sqrt/1
  Sqrt/1 -> Divide/2
  Gain/1 -> Divide/1

== system CompleteEngineModel_turbo/Engine/Turbocharger/Turbine/PiT ==
  p_em : Inport
  p_es : Inport  Port=2
  MinMax : MinMax  Inputs=2
  Product4 : Product  Inputs=*/  RndMeth=Zero
  one1 : Constant
  PiT : Outport
  wires:
  Product4/1 -> MinMax/1
  one1/1 -> MinMax/2
  p_em/1 -> Product4/2
  MinMax/1 -> PiT/1  "PiT"
  p_es/1 -> Product4/1

== system CompleteEngineModel_turbo/Engine/Turbocharger/Turbine/TFP2Wt ==
  p_em [Pa] : Inport
  TFP : Inport  Port=2
  T_em : Inport  Port=3
  Divide : Product  Inputs=*/
  Product : Product
  Sqrt : Sqrt  SaturateOnIntegerOverflow=on
  m_dot_t : Outport
  wires:
  p_em [Pa]/1 -> Product/2
  T_em/1 -> Sqrt/1
  TFP/1 -> Product/1
  Divide/1 -> m_dot_t/1
  Product/1 -> Divide/1
  Sqrt/1 -> Divide/2

== system CompleteEngineModel_turbo/Engine/Turbocharger/Turbine/TFPmod ==
  PiT : Inport
  Constant : Constant  Value=k_1
  Constant1 : Constant
  Gain : Gain  Gain=k_0
  "Pa -> kPa" : Gain  Gain=1/1000
  Power : Math  Operator=pow  SaturateOnIntegerOverflow=on
  Sqrt : Sqrt  SaturateOnIntegerOverflow=on
  Sum : Sum  Inputs=+-|
  TFPmod : Outport
  wires:
  PiT/1 -> Power/1
  Constant/1 -> Power/2
  Power/1 -> Sum/2
  Constant1/1 -> Sum/1
  Sum/1 -> Sqrt/1
  Sqrt/1 -> Gain/1
  Gain/1 -> "Pa -> kPa"/1
  "Pa -> kPa"/1 -> TFPmod/1

== system CompleteEngineModel_turbo/Engine/Turbocharger/Turbine/Tq_t ==
  m_dot_t : Inport
  T_em : Inport  Port=2
  T04 : Inport  Port=3
  w_tc : Inport  Port=4
  Constant : Constant  Value=cp_exh
  Divide : Product  Inputs=*/
  Product : Product  Inputs=3
  Sum : Sum  Inputs=|+-
  Tq_t : Outport
  wires:
  Divide/1 -> Tq_t/1
  Constant/1 -> Product/2
  Product/1 -> Divide/1
  Sum/1 -> Product/3
  w_tc/1 -> Divide/2
  m_dot_t/1 -> Product/1
  T_em/1 -> Sum/1
  T04/1 -> Sum/2

== system CompleteEngineModel_turbo/Engine/Turbocharger/Turbine/Tt ==
  T_em : Inport
  etaT : Inport  Port=2
  PiT : Inport  Port=3
  Constant : Constant  Value=(gamma_exh - 1) / gamma_exh
  Constant1 : Constant
  Power : Math  Operator=pow  SaturateOnIntegerOverflow=on
  Product : Product
  Product1 : Product
  Sum : Sum  Inputs=+-|
  Sum1 : Sum  Inputs=+-|
  T04 : Outport
  wires:
  T_em/1 -> Product1/2
  etaT/1 -> Product/2
  Product1/1 -> T04/1
  Power/1 -> Sum/2
  Constant/1 -> Power/2
  Constant1/1 -> Sum1/1, Sum/1
  PiT/1 -> Power/1
  Sum/1 -> Product/1
  Product/1 -> Sum1/2
  Sum1/1 -> Product1/1

== system CompleteEngineModel_turbo/Engine/Turbocharger/Turbine/etaT ==
  BSR : Inport
  Constant : Constant  Value=etaTmin
  Constant1 : Constant  Value=BSR_max
  Constant2 : Constant
  Divide : Product  Inputs=*/
  Gain : Gain  Gain=eta_t_max
  Max : MinMax  Function=max  Inputs=2
  Square : Math  Operator=square  SaturateOnIntegerOverflow=on
  Sum : Sum  Inputs=|+-
  Sum1 : Sum  Inputs=+-|
  etaT : Outport
  wires:
  Max/1 -> etaT/1
  Constant/1 -> Max/2
  BSR/1 -> Sum/1
  Gain/1 -> Max/1
  Constant1/1 -> Sum/2, Divide/2
  Sum/1 -> Divide/1
  Divide/1 -> Square/1
  Square/1 -> Sum1/2
  Constant2/1 -> Sum1/1
  Sum1/1 -> Gain/1

== system CompleteEngineModel_turbo/Engine/Turbocharger/Wastegate/Psi(PI) ==
  PI : Inport
  (g+1)/g : Constant  Value=(gamma_air+1)/gamma_air
  2/g : Constant  Value=2/gamma_air
  2g/(g-1) : Constant  Value=(2*gamma_air)/(gamma_air-1)
  Math Function : Math  Operator=pow  SignedPower=on  SaturateOnIntegerOverflow=on
  Math Function1 : Math  Operator=pow  SignedPower=on  SaturateOnIntegerOverflow=on
  MinMax : MinMax  Function=max  Inputs=2
  PI critical (2/(g+1))^(g/(g-1)) : Constant  Value=(2/(gamma_air+1))^(gamma_air/(gamma_air-1))
  Product : Product  RndMeth=Zero
  Sqrt : Sqrt  AlgorithmType=Newton-Raphson  SaturateOnIntegerOverflow=on
  Subtract : Sum  Inputs=+-
  "[0,1]" : Saturate  UpperLimit=1  LowerLimit=0
  Psi : Outport
  wires:
  PI/1 -> "[0,1]"/1  "PI"
  PI critical (2/(g+1))^(g/(g-1))/1 -> MinMax/2
  MinMax/1 -> Math Function/1, Math Function1/1  "PIlim"
  2/g/1 -> Math Function/2
  (g+1)/g/1 -> Math Function1/2
  "[0,1]"/1 -> MinMax/1
  Math Function/1 -> Subtract/1
  Math Function1/1 -> Subtract/2
  Subtract/1 -> Product/1
  2g/(g-1)/1 -> Product/2
  Product/1 -> Sqrt/1
  Sqrt/1 -> Psi/1  "Psi"

== system CompleteEngineModel_turbo/ECU/Boost Control/Throttle Feed Forward /Cylinder air flow REF/Volymetrisk effektivitet ==
  " p_im" : Inport
  N : Inport  Port=2
  Abs : Abs
  Abs1 : Abs
  Sqrt : Sqrt  SaturateOnIntegerOverflow=on
  Sqrt1 : Sqrt  SaturateOnIntegerOverflow=on
  Sum : Sum  Inputs=|++
  Sum1 : Sum  Inputs=|++
  c0 : Constant  Value=Intake_mainfold_const(1)
  c1 : Gain  Gain=Intake_mainfold_const(2)
  c2 : Gain  Gain=Intake_mainfold_const(3)
  eta_vol : Outport
  wires:
  Sum1/1 -> eta_vol/1
  Abs/1 -> Sqrt/1
  Abs1/1 -> Sqrt1/1
  c2/1 -> Sum/2
  Sqrt/1 -> c1/1
  c0/1 -> Sum1/2
  c1/1 -> Sum/1
  Sqrt1/1 -> c2/1
  Sum/1 -> Sum1/1
  " p_im"/1 -> Abs/1
  N/1 -> Abs1/1

== system CompleteEngineModel_turbo/ECU/Boost Control/Throttle Feed Forward /Cylinder air flow REF/m_dot_ac_system ==
  p_im_REF : Inport
  Eta_vol_REF : Inport  Port=2
  N : Inport  Port=3
  Divide : Product  Inputs=*/
  Product : Product  Inputs=5
  Product1 : Product  Inputs=3
  R : Constant  Value=R_air
  T_01 : Constant  Value=T01
  V_d : Constant  Value=V_d
  n_cyl : Constant  Value=n_cyl
  n_r : Constant  Value=n_r
  m_dot_ac : Outport
  wires:
  V_d/1 -> Product/3
  n_cyl/1 -> Product/4
  Product/1 -> Divide/1
  n_r/1 -> Product1/1
  T_01/1 -> Product1/2
  R/1 -> Product1/3
  Product1/1 -> Divide/2
  Divide/1 -> m_dot_ac/1
  p_im_REF/1 -> Product/1
  N/1 -> Product/2
  Eta_vol_REF/1 -> Product/5
